simulink model "disturbances_report_sim"  (R2023b)
settings: Solver=ode5  StartTime=0.0  StopTime=5643.69  FixedStep=1  RelTol=1e-3
values from neighbouring files (symbols this model uses):
  A = [0.49 0.49 0.49 0.49 0.49 0.49 0.49 0.49 0.49 0.49 0.49 0.49 0.49 0.49]    [disturbances_report.m]    (also in sat_dist.m = [6*1e-2; 6*1e-2; 6*1e-2; 6*1e-2; 4*1e-2; 4*1e-2; 12*1e-2; 12)
  a = 1 / ( (2/r) - (v^2 / mu) )    [car2par.m]    (also in disturbances_report.m = 6851.22197053)
  c1 = [1 - rho_s; 1 - rho_s; 1 - rho_s]    [disturbances_report.m]
  CD = 2.2    [disturbances_report.m]
  d0 = 1.585*10^-12    (= 1.585e-12)    [disturbances_report.m]
  e = norm(ee)    [car2par.m]    (also in disturbances_report.m = 0.00183012221618)
  H = 60.828    [disturbances_report.m]
  h0 = 450    [disturbances_report.m]
  i = rad2deg(i)    [car2par.m]    (also in disturbances_report.m = 1.69998086203)
  I_ext = diag([I1_ext I2_ext I3_ext])    [disturbances_report.m]
  Iinv_ext = I_ext\eye(3)    [disturbances_report.m]
  jb = [0.01; 0.05; 0.01]    [disturbances_report.m]    (also in sat_dist.m)
  muE = astroConstants(13)    [disturbances_report.m]
  N = [1 0 0]'    [car2par.m]    (also in disturbances_report.m = [0 1 0; 0 -1 0; sqrt(2)/2 0 sqrt(2)/2; -sqrt(2)/2 0 sqrt(2)/; sat_dist.m = [1 0 0; 0 1 0; -1 0 0; 0 -1 0; 0 0 1; 0 0 -1; 1 0 0; -1 0 0;)
  n_sun = sqrt(mu_sun/a_E^3)    [disturbances_report.m]
  nn = sqrt(muE/a^3)    [disturbances_report.m]
  om = rad2deg(om)    [car2par.m]    (also in disturbances_report.m = 1.77284810319)
  OM = rad2deg(OM)    [car2par.m]    (also in disturbances_report.m = 0.55426850949)
  omega0 = zeros(3,1)    [disturbances_report.m]    (also in sat_dist.m = [0; 0; n])
  omegaE = deg2rad(15)/3600    [disturbances_report.m]    (also in sat_dist.m)
  onesM = ones(3, n)    [disturbances_report.m]
  onesV = ones(n,1)    [disturbances_report.m]
  P = astroConstants(31)/(astroConstants(5)*10^3)    [disturbances_report.m]    (also in sat_dist.m = Fe/c)
  r_Fskew = zeros(n*3, n*3)    [disturbances_report.m]
  rho_d = [0.1 0.1 0.1 0.1 0.1 0.1 0.1 0.1 0.1 0.1 0.1 0.1 0.1 0.1]    [disturbances_report.m]
  rho_s = [0.5 0.5 0.5 0.5 0.5 0.5 0.1 0.1 0.1 0.1 0.1 0.1 0.1 0.1]    [disturbances_report.m]
  Rt = astroConstants(23)    [disturbances_report.m]    (also in sat_dist.m)
  s0 = zeros(3,1)    [disturbances_report.m]    (also in sat_dist.m)
  th_0 = 0    [disturbances_report.m]
  tol = 0.2    [disturbances_report.m]
undefined symbols (not defined in the file or in its folder): gh, magnitude
libraries: matrix_library x6, simulink x4, simulink_extras x1, dspmathops x1
(part 2 of 2)

== system disturbances_report_sim/Kinematics/Kinematics 313/s_313 - A/R1 ==
  x : Inport
  Constant : Constant  Value=[1; 0; 0]
  Constant1 : Constant  Value=0
  Cos : Trigonometry  Operator=cos
  Gain : Gain  Gain=-1
  Matrix Concatenate : Concatenate  NumInputs=3  Mode=Multidimensional array  ConcatenateDimension=2
  Sin : Trigonometry
  Vector Concatenate : Concatenate  NumInputs=3
  Vector Concatenate1 : Concatenate  NumInputs=3
  R1 : Outport
  wires:
  Sin/1 -> Gain/1, Vector Concatenate/2
  Gain/1 -> Vector Concatenate1/3
  Cos/1 -> Vector Concatenate1/2, Vector Concatenate/3
  Constant1/1 -> Vector Concatenate1/1, Vector Concatenate/1
  Vector Concatenate/1 -> Matrix Concatenate/3
  Constant/1 -> Matrix Concatenate/1
  Vector Concatenate1/1 -> Matrix Concatenate/2
  x/1 -> Sin/1, Cos/1
  Matrix Concatenate/1 -> R1/1

== system disturbances_report_sim/Kinematics/Kinematics 313/s_313 - A/R3_1 ==
  x : Inport
  Constant : Constant  Value=[0; 0; 1]
  Constant1 : Constant  Value=0
  Cos : Trigonometry  Operator=cos
  Gain : Gain  Gain=-1
  Matrix Concatenate : Concatenate  NumInputs=3  Mode=Multidimensional array  ConcatenateDimension=2
  Sin : Trigonometry
  Vector Concatenate : Concatenate  NumInputs=3
  Vector Concatenate1 : Concatenate  NumInputs=3
  R3 : Outport
  wires:
  Matrix Concatenate/1 -> R3/1
  Constant1/1 -> Vector Concatenate1/3, Vector Concatenate/3
  x/1 -> Cos/1, Sin/1
  Vector Concatenate1/1 -> Matrix Concatenate/2
  Gain/1 -> Vector Concatenate/2
  Constant/1 -> Matrix Concatenate/3
  Cos/1 -> Vector Concatenate/1, Vector Concatenate1/2
  Sin/1 -> Gain/1, Vector Concatenate1/1
  Vector Concatenate/1 -> Matrix Concatenate/1

== system disturbances_report_sim/Kinematics/Kinematics 313/s_313 - A/R3_2 ==
  x : Inport
  Constant : Constant  Value=[0; 0; 1]
  Constant1 : Constant  Value=0
  Cos : Trigonometry  Operator=cos
  Gain : Gain  Gain=-1
  Matrix Concatenate : Concatenate  NumInputs=3  Mode=Multidimensional array  ConcatenateDimension=2
  Sin : Trigonometry
  Vector Concatenate : Concatenate  NumInputs=3
  Vector Concatenate1 : Concatenate  NumInputs=3
  R3 : Outport
  wires:
  Vector Concatenate/1 -> Matrix Concatenate/1
  Sin/1 -> Vector Concatenate1/1, Gain/1
  Cos/1 -> Vector Concatenate1/2, Vector Concatenate/1
  Constant/1 -> Matrix Concatenate/3
  Gain/1 -> Vector Concatenate/2
  Vector Concatenate1/1 -> Matrix Concatenate/2
  x/1 -> Sin/1, Cos/1
  Constant1/1 -> Vector Concatenate/3, Vector Concatenate1/3
  Matrix Concatenate/1 -> R3/1

== matlab function disturbances_report_sim/Subsystem/Magnetic Field/MATLAB Function ==
  data: r input; B output; theta input; phi input; gh input
function B = calculateField(r, theta, phi, gh)

N = 13;         % Order of the field
lat = pi/2 - theta;
lon = phi;

R = 6371.2;     % Radius of Earth in IGRF
ratio = R / r;

sin_lat = sin(lat);
cos_lat = cos(lat);
sin_lon = sin(lon);
cos_lon = cos(lon);

npq = (N * (N+3)) / 2;

p = zeros(npq, 1);
p(1) = 2*sin_lat;
p(2) = 2*cos_lat;
p(3) = 4.5*sin_lat^2 - 1.5;
p(4) = 3*sqrt(3) * cos_lat * sin_lat;

q = zeros(npq, 1);
q(1) = -cos_lat;
q(2) = sin_lat;
q(3) = -3 * cos_lat * sin_lat;
q(4) = sqrt(3) * (sin_lat^2 - cos_lat^2);

sl = zeros(N+1, 1);
sl(1) = sin_lon;

cl = zeros(N+1, 1);
cl(1) = cos_lon;

Bx = 0; By = 0; Bz = 0;
l = 1; n = 0; m = 1;
fn = nan; rr = nan;

for k = 1:npq

    if n < m
        m = 0;
        n = n + 1;
        rr = ratio^(n+2);
        fn = n;
    end

    fm = m;

    if k >= 5

        if m == n
            a = sqrt(1 - 0.5/fm);
            j = k - n - 1;
            p(k) = (1 + 1/fm) * a * cos_lat * p(j);
            q(k) = a * (cos_lat * q(j) + sin_lat/fm * p(j));
            sl(m) = sl(m-1)*cl(1) + cl(m-1)*sl(1);
            cl(m) = cl(m-1)*cl(1) - sl(m-1)*sl(1);
        else
            a = sqrt(fn^2 - fm^2);
            b = sqrt((fn-1)^2 - fm^2) / a;
            c = (2*fn - 1) / a;
            ii = k - n;
            j = k - 2*n + 1;
            p(k) = (fn+1) * (c * sin_lat/fn * p(ii) - b/(fn-1) * p(j));
            q(k) = c * (sin_lat * q(ii) - cos_lat/fn * p(ii)) - b * q(j);
        end

    end

    a = rr * gh(l);
    
    if m == 0

        Bx = Bx + a*q(k);
        Bz = Bz - a*p(k);
        
        l = l + 1;

    else
        
        b = rr * gh(l+1);
        c = a*cl(m) + b*sl(m);
        Bx = Bx + c * q(k);
        Bz = Bz - c * p(k);
        
        if cos_lat > 0
            By = By + (a*sl(m) - b*cl(m)) * fm * p(k)/((fn+1) * cos_lat);
        else
            By = By + (a*sl(m) - b*cl(m)) * q(k) * sin_lat;
        end
        
        l = l + 2;

    end

    m = m + 1;

end

B_NED = [Bx; By; Bz] * 1e-9;

% Convert NED to ECEF
R = [-sin_lat * cos_lon,    -sin_lon,   -cos_lat * cos_lon;
     -sin_lat * sin_lon,    cos_lon,    -cos_lat * sin_lon;
     cos_lat,               0,          -sin_lat            ];

B = R * B_NED;
